simulink model "power_rectifier_ideal"  (Simulink 6.0)
settings: Solver=ode15s  SolverMode=SingleTasking  StartTime=0.0  StopTime=0.1  RelTol=1e-3
libraries: powerlib x16, powerlib_extras x1
settings Model: Creator=sybille  LastModifiedBy=batserve  ExtModeTrigMode=oneshot  ExtModeArmWhenConnect=off  ExtModeAutoUpdateStatusClock=off
settings DataIOCC: LimitDataPoints=off  SaveOutput=off  SaveTime=off  SignalLoggingName=sigsOut
settings OptimizationCC: BlockReduction=off  BooleanDataType=off
settings DebuggingCC: SolverPrmCheckMsg=none  UnconnectedInputMsg=none  UnconnectedOutputMsg=none
settings HardwareCC: TargetUnknown=on
settings RTWCC: TemplateMakefile=grt_unix.tmf

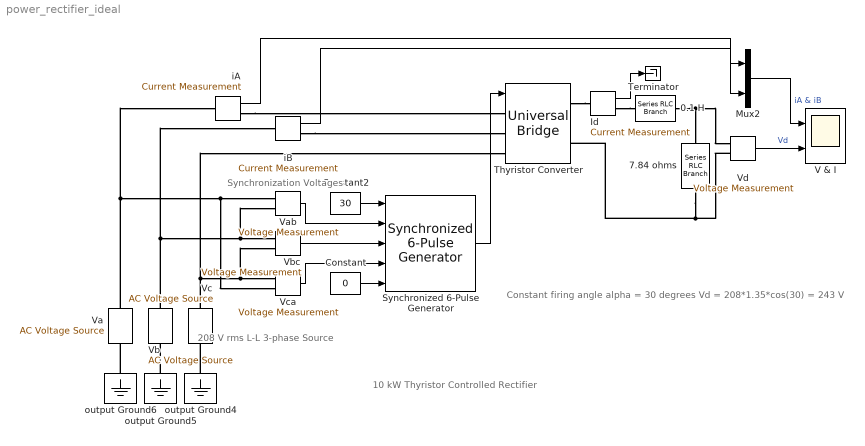
== system power_rectifier_ideal ==
  note: Synchronization Voltages
  note: 208 V rms L-L
      | 3-phase Source
  note: 10 kW Thyristor Controlled Rectifier
  note: Constant firing angle alpha = 30 degrees
      | Vd = 208*1.35*cos(30) = 243 V
  0.1 H : powerlib/Elements/Series RLC Branch  PhysicalDomain=powersysdomain  SubClassName=unknown  LeftPortType=p1  RightPortType=p1  LConnTagsString=__new0  RConnTagsString=__new0  Resistance=0  Inductance=100e-3  Capacitance=inf  Measurements=None
  7.84 ohms : powerlib/Elements/Series RLC Branch  Orientation=down  PhysicalDomain=powersysdomain  SubClassName=unknown  LeftPortType=p1  RightPortType=p1  LConnTagsString=__new0  RConnTagsString=__new0  Resistance=7.84  Inductance=0  Capacitance=inf  Measurements=None
  Constant : Constant  Value=0
  Constant2 : Constant  Value=30
  Id : powerlib/Measurements/Current Measurement  Tag=PoWeRsYsTeMmEaSuReMeNt  PhasorSimulation=off  OutputType=Magnitude  PSBequivalent=0
  Mux2 : Mux  Inputs=2
  Synchronized 6-Pulse Generator : powerlib_extras/Control  Blocks/Synchronized 6-Pulse Generator  freq=60  pwidth=10  Double_Pulse=off
  Terminator : Terminator
  Thyristor Converter : powerlib/Power Electronics/Universal Bridge  Arms=3  SnubberResistance=500  SnubberCapacitance=.01e-6  Device=Thyristors  Ron=0.01  Lon=1e-6  ForwardVoltages="[  0.8  0.8  ]"  ForwardVoltage=0.8  GTOparameters=[ 10e-6 , 20e-6 ]  IGBTparameters=[ 1e-6 , 2e-6 ]  Measurements=Device currents
  V & I : Scope  NumInputPorts=2
      settings: TimeRange=0.1  YMin=-40~0  YMax=40~250  DataFormat=Structure
  Va : powerlib/Electrical Sources/AC Voltage Source  Description=source block  Orientation=up  Amplitude=208*sqrt(2/3)  Phase=0  Frequency=60  SampleTime=0  Measurements=None
      settings: AttributesFormatString=\n
  Vab : powerlib/Measurements/Voltage Measurement  Tag=PoWeRsYsTeMmEaSuReMeNt  PhasorSimulation=off  OutputType=Magnitude  PSBequivalent=0
  Vb : powerlib/Electrical Sources/AC Voltage Source  Description=source block  Orientation=up  Amplitude=208*sqrt(2/3)  Phase=-120  Frequency=60  SampleTime=0  Measurements=None
      settings: AttributesFormatString=\n
  Vbc : powerlib/Measurements/Voltage Measurement  Tag=PoWeRsYsTeMmEaSuReMeNt  PhasorSimulation=off  OutputType=Magnitude  PSBequivalent=0
  Vc : powerlib/Electrical Sources/AC Voltage Source  Description=source block  Orientation=up  Amplitude=208*sqrt(2/3)  Phase=120  Frequency=60  SampleTime=0  Measurements=None
      settings: AttributesFormatString=\n
  Vca : powerlib/Measurements/Voltage Measurement  Tag=PoWeRsYsTeMmEaSuReMeNt  PhasorSimulation=off  OutputType=Magnitude  PSBequivalent=0
  Vd : powerlib/Measurements/Voltage Measurement  Tag=PoWeRsYsTeMmEaSuReMeNt  PhasorSimulation=off  OutputType=Magnitude  PSBequivalent=0
  iA : powerlib/Measurements/Current Measurement  Tag=PoWeRsYsTeMmEaSuReMeNt  PhasorSimulation=off  OutputType=Magnitude  PSBequivalent=0
  iB : powerlib/Measurements/Current Measurement  Tag=PoWeRsYsTeMmEaSuReMeNt  PhasorSimulation=off  OutputType=Magnitude  PSBequivalent=0
  output Ground4 : powerlib/Elements/Ground  Orientation=down  PhysicalDomain=powersysdomain  SubClassName=unknown  LeftPortType=p1  RightPortType=p1  LConnTagsString=a
  output Ground5 : powerlib/Elements/Ground  Orientation=down  PhysicalDomain=powersysdomain  SubClassName=unknown  LeftPortType=p1  RightPortType=p1  LConnTagsString=a
  output Ground6 : powerlib/Elements/Ground  Orientation=down  PhysicalDomain=powersysdomain  SubClassName=unknown  LeftPortType=p1  RightPortType=p1  LConnTagsString=a
  wires:
  Constant/1 -> Synchronized 6-Pulse Generator/5
  Constant2/1 -> Synchronized 6-Pulse Generator/1
  Mux2/1 -> V & I/1  "iA & iB"
  Vca/1 -> Synchronized 6-Pulse Generator/4
  Vbc/1 -> Synchronized 6-Pulse Generator/3
  Vab/1 -> Synchronized 6-Pulse Generator/2
  Synchronized 6-Pulse Generator/1 -> Thyristor Converter/1
  iA/1 -> Mux2/1
  iB/1 -> Mux2/2
  Vd/1 -> V & I/2  "Vd"
  Id/1 -> Terminator/1
  connections:
  Thyristor Converter/RConn1 -- Id/LConn1
  Vd/LConn2 -- Thyristor Converter/RConn2 -- 7.84 ohms/RConn1
  iA/RConn1 -- Thyristor Converter/LConn1
  iB/RConn1 -- Thyristor Converter/LConn2
  Vc/RConn1 -- Vca/LConn1 -- Vbc/LConn2 -- Thyristor Converter/LConn3
  Vb/RConn1 -- Vbc/LConn1 -- Vab/LConn2 -- iB/LConn1
  Va/RConn1 -- Vab/LConn1 -- Vca/LConn2 -- iA/LConn1
  Id/RConn1 -- 0.1 H/LConn1
  output Ground6/LConn1 -- Va/LConn1
  output Ground5/LConn1 -- Vb/LConn1
  output Ground4/LConn1 -- Vc/LConn1
  0.1 H/RConn1 -- 7.84 ohms/LConn1 -- Vd/LConn1
